simulink model "DC_MOTOR_CONTROL"  (R2022b)
settings: Solver=FixedStepAuto  StartTime=0.0  StopTime=100  FixedStep=0.01  RelTol=1e-3
libraries: fod x4, arduinolib x3, arduinosensorlib x1, SignalEditorBlockLib x1, simulink x1
settings Model: SimulationMode=external  ExtModeTrigDuration=2  Creator=Mario  LastModifiedBy=mario
settings DataIOCC: ReturnWorkspaceOutputs=off
settings OptimizationCC: EnhancedBackFolding=on  PassReuseOutputArgsThreshold=0  MaxStackSize=64  OptimizeBlockOrder=speed  DifferentSizesBufferReuse=on  OptimizationCustomize=off
settings DebuggingCC: ParameterTunabilityLossMsg=error
settings HardwareCC: ProdBitPerPointer=32  ProdBitPerSizeT=32  ProdBitPerPtrDiffT=32  ProdLargestAtomicInteger=Long  ProdLargestAtomicFloat=Double  ProdWordSize=32  ProdHWDeviceType=ARM Compatible->ARM Cortex  UseEmbeddedCoderFeatures=off
settings SFSimCC: MATLABDynamicMemAlloc=off
settings RTWCC: Description=Embedded Coder  SystemTargetFile=ert.tlc  HardwareBoard=Arduino Due  TLCOptions=-aInlineSetEventsForThisBaseRateFcn=TLC_FALSE -aSuppressMultiTaskScheduler=TLC_FALSE -aRateBasedStepFcn=1  TemplateMakefile=ert_default_tmf  Toolchain=Arduino ARM  BuildConfiguration=Faster Runs
settings CodeAppCC: ForceParamTrailComments=on  OperatorAnnotations=on
settings ERTTargetCC: ERTCustomFileBanners=off  SupportContinuousTime=on  SupportNonInlinedSFcns=on  RemoveResetFunc=off  SupportVariableSizeSignals=on  ModelStepFunctionPrototypeControlCompliant=off  ExtModeTransport=3  ExtModeStaticAlloc=on  ExtModeAutomaticAllocSize=off  ExtModeStaticAllocSize=24576  ExtModeMexFile=ext_xcp  ExtModeIntrfLevel=Level2 - Open

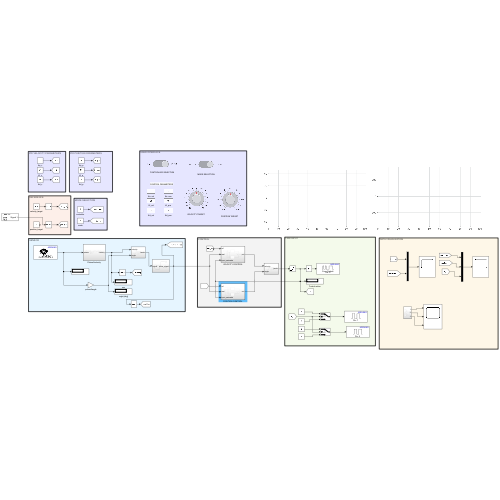
[thumbnail: Simulink's stored preview of the top-level diagram]
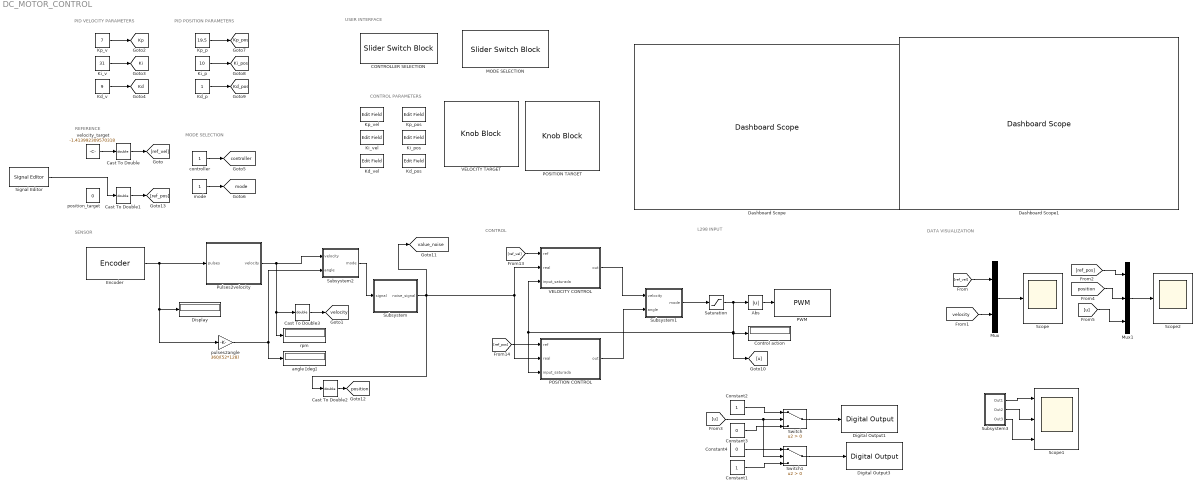
== system DC_MOTOR_CONTROL ==
  note: CONTROL PARAMETERS
  note: USER INTERFACE
  note: CONTROL
  note: MODE SELECTION
  note: DATA VISUALIZATION
  note: PID VELOCITY PARAMETERS
  note: SENSOR
  note: REFERENCE
  note: L298 INPUT
  note: PID POSITION PARAMETERS
  Abs : Abs  SaturateOnIntegerOverflow=off
  CONTROLLER SELECTION : SliderSwitchBlock  LabelPosition=Hide
      settings: Values={{'PID', 'FOPID'}, [0 1]}
  Cast To Double{,1..3} (4 alike) : DataTypeConversion  OutDataTypeStr=double  SaturateOnIntegerOverflow=off  RndMeth=Floor
  Constant1 : Constant
  Constant2 : Constant
  Constant3 : Constant  Value=0
  Constant4 : Constant  Value=0
  Control action : Display
  Dashboard Scope : DashboardScope  Ymin=-70  Ymax=70  UpdateMode=Scroll
  Dashboard Scope1 : DashboardScope  Ymin=-360  Ymax=360  UpdateMode=Scroll
  Digital Output1 : arduinolib/Digital Output  pinNumber=7  Direction=output  blockPlatform=arduino
  Digital Output3 : arduinolib/Digital Output  pinNumber=5  Direction=output  blockPlatform=arduino
  Display : Display
  Encoder : arduinosensorlib/Encoder  InputA=3  InputB=2  Mode=No reset  SampleTime=-1
  Kd_p : Constant
  Kd_pos : EditField  LabelPosition=Hide  ShowInitialText=on  Alignment=Center
  Kd_v : Constant  Value=9
  Kd_vel : EditField  LabelPosition=Hide  ShowInitialText=on  Alignment=Center
  Ki_p : Constant  Value=10
  Ki_pos : EditField  LabelPosition=Hide  ShowInitialText=on  Alignment=Center
  Ki_v : Constant  Value=31
  Ki_vel : EditField  LabelPosition=Hide  ShowInitialText=on  Alignment=Center
  Kp_p : Constant  Value=19.5
  Kp_pos : EditField  LabelPosition=Hide  ShowInitialText=on  Alignment=Center
  Kp_v : Constant  Value=7
  Kp_vel : EditField  LabelPosition=Hide  ShowInitialText=on  Alignment=Center
  MODE SELECTION : SliderSwitchBlock  LabelPosition=Hide
      settings: Values={{'Velocity', 'Position'}, [0 1]}
  Mux : Mux  Inputs=2
  Mux1 : Mux  Inputs=3
  POSITION CONTROL : Subsystem
  POSITION TARGET : KnobBlock  LabelPosition=Hide  ScaleMin=-360  ScaleMax=360
  PWM : arduinolib/PWM  pinNumber=8  frequencyType=Default  desiredFrequency=490.2  achievableFrequency=490.2
  Pulses2velocity : Subsystem
  Saturation : Saturate  UpperLimit=255  LowerLimit=-255
  Scope : Scope
  Scope1 : Scope  NumInputPorts=3
  Scope2 : Scope
  Signal Editor : SignalEditorBlockLib/Signal Editor  FileName=ANGLE_REFERENCE.mat  ActiveScenario=Scenario  ActiveSignal=Signal 1  IsBus=off  OutputBusObjectStr=Bus: BusObject  SampleTime=0  Interpolate=off  ZeroCross=off  OutputAfterFinalValue=Setting to zero  Unit=inherit  PreserveSignalName=on
  Subsystem : Subsystem
  Subsystem1 : Subsystem
  Subsystem2 : Subsystem
  Subsystem3 : Subsystem
  Switch : Switch  Criteria=u2 > Threshold  SaturateOnIntegerOverflow=off  InputSameDT=off
  Switch1 : Switch  Criteria=u2 > Threshold  SaturateOnIntegerOverflow=off  InputSameDT=off
  VELOCITY CONTROL : Subsystem
  VELOCITY TARGET : KnobBlock  LabelPosition=Hide  ScaleMin=-70  ScaleMax=70
  angle [deg] : Display
  controller : Constant
  mode : Constant
  position_target : Constant  Value=0
  pulses2angle : Gain  Gain=360/(52*128)
  rpm : Display
  velocity_target : Constant  Value=-1.413992309570318
  tag scope: Kd=global, Kd_pos=global, Ki=global, Ki_pos=global, Kp=global, Kp_pos=global, controller=global, mode=global, position=global, value_noise=global, velocity=global
  wires:
  Constant3/1 -> Switch/3
  Constant2/1 -> Switch/1
  Switch/1 -> Digital Output1/1
  Switch1/1 -> Digital Output3/1
  Pulses2velocity/1(velocity) -> Subsystem2/1(velocity), rpm/1, Cast To Double3/1
  velocity_target/1 -> Cast To Double/1
  Encoder/1 -> Pulses2velocity/1(pulses), pulses2angle/1, Display/1
  Saturation/1 -> POSITION CONTROL/3(input_saturada), VELOCITY CONTROL/3(input_saturada), [u], Control action/1, Abs/1
  Constant4/1 -> Switch1/1
  Constant1/1 -> Switch1/3
  [ref_vel] -> Mux/1
  [velocity] -> Mux/2
  Kp_v/1 -> [Kp]
  Ki_v/1 -> [Ki]
  Kd_v/1 -> [Kd]
  controller/1 -> [controller]
  mode/1 -> [mode]
  VELOCITY CONTROL/1(out) -> Subsystem1/1(velocity)
  POSITION CONTROL/1(out) -> Subsystem1/2(angle)
  pulses2angle/1 -> Subsystem2/2(angle), angle [deg]/1
  Kp_p/1 -> [Kp_pos]
  Kd_p/1 -> [Kd_pos]
  Ki_p/1 -> [Ki_pos]
  Mux/1 -> Scope/1
  Abs/1 -> PWM/1
  [u] -> Switch/2, Switch1/2
  Subsystem2/1(mode) -> Subsystem/1(signal)
  [ref_vel] -> VELOCITY CONTROL/1(ref)
  [ref_pos] -> POSITION CONTROL/1(ref)
  Subsystem3/1(Out1) -> Scope1/1
  Subsystem3/2(Out2) -> Scope1/2
  Subsystem3/3(Out3) -> Scope1/3
  Subsystem/1(noise_signal) -> Cast To Double2/1, POSITION CONTROL/2(real), VELOCITY CONTROL/2(real), [value_noise]
  Mux1/1 -> Scope2/1
  [ref_pos] -> Mux1/1
  [position] -> Mux1/2
  Cast To Double/1 -> [ref_vel]
  Cast To Double1/1 -> [ref_pos]
  Cast To Double2/1 -> [position]
  Cast To Double3/1 -> [velocity]
  Signal Editor/1 -> Cast To Double1/1
  [u] -> Mux1/3
  Subsystem1/1(mode) -> Saturation/1

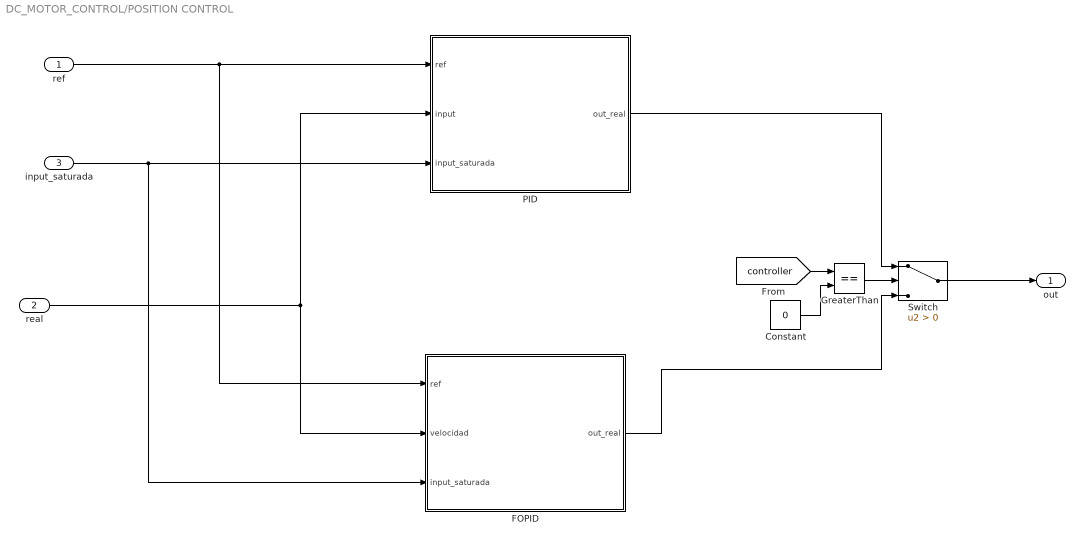
== system DC_MOTOR_CONTROL/POSITION CONTROL ==
  ref : Inport
  real : Inport  Port=2
  input_saturada : Inport  Port=3
  Constant : Constant  Value=0
  "FOPID " : Subsystem
  GreaterThan : RelationalOperator  Operator===  OutDataTypeStr=boolean  RndMeth=Simplest  InputSameDT=off
  PID : Subsystem
  Switch : Switch  Criteria=u2 > Threshold  SaturateOnIntegerOverflow=off  InputSameDT=off
  out : Outport
  wires:
  input_saturada/1 -> "FOPID "/3(input_saturada), PID/3(input_saturada)
  ref/1 -> "FOPID "/1(ref), PID/1(ref)
  real/1 -> "FOPID "/2(velocidad), PID/2(input)
  "FOPID "/1(out_real) -> Switch/3
  PID/1(out_real) -> Switch/1
  Switch/1 -> out/1
  [controller] -> GreaterThan/1
  Constant/1 -> GreaterThan/2
  GreaterThan/1 -> Switch/2

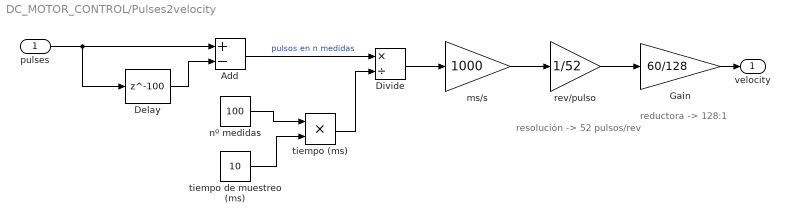
== system DC_MOTOR_CONTROL/Pulses2velocity ==
  note: reductora -> 128:1
  note: resolución -> 52 pulsos/rev
  pulses : Inport
  Add : Sum  Inputs=+-
  Delay : Delay  DelayLength=100
  Divide : Product  Inputs=*/
  Gain : Gain  Gain=60/128
  ms/s : Gain  Gain=1000
  nº medidas : Constant  Value=100
  rev/pulso : Gain  Gain=1/52
  tiempo (ms) : Product  Inputs=**
  tiempo de muestreo (ms) : Constant  Value=10
  velocity : Outport
  wires:
  Delay/1 -> Add/2
  Divide/1 -> ms/s/1
  pulses/1 -> Delay/1, Add/1
  nº medidas/1 -> tiempo (ms)/1
  Add/1 -> Divide/1  "pulsos en n medidas"
  rev/pulso/1 -> Gain/1
  Gain/1 -> velocity/1
  ms/s/1 -> rev/pulso/1
  tiempo de muestreo (ms)/1 -> tiempo (ms)/2
  tiempo (ms)/1 -> Divide/2

== system DC_MOTOR_CONTROL/Subsystem ==
  signal : Inport
  Band-Limited White Noise : simulink/Sources/Band-Limited White Noise  Cov=0  Ts=0.01  seed=[23341]
  Sum : Sum  Inputs=|++
  noise_signal : Outport
  wires:
  Sum/1 -> noise_signal/1
  signal/1 -> Sum/2
  Band-Limited White Noise/1 -> Sum/1

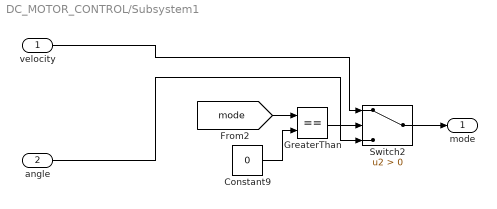
== system DC_MOTOR_CONTROL/Subsystem1 ==
  velocity : Inport
  angle : Inport  Port=2
  Constant9 : Constant  Value=0
  GreaterThan : RelationalOperator  Operator===  OutDataTypeStr=boolean  RndMeth=Simplest  InputSameDT=off
  Switch2 : Switch  Criteria=u2 > Threshold  SaturateOnIntegerOverflow=off  InputSameDT=off
  mode : Outport
  wires:
  [mode] -> GreaterThan/1
  GreaterThan/1 -> Switch2/2
  Switch2/1 -> mode/1
  Constant9/1 -> GreaterThan/2
  velocity/1 -> Switch2/1
  angle/1 -> Switch2/3

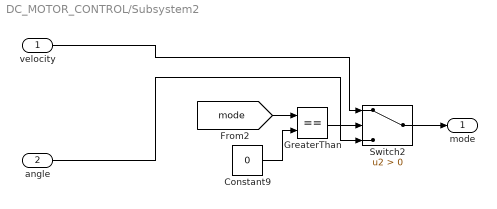
== system DC_MOTOR_CONTROL/Subsystem2 ==
  velocity : Inport
  angle : Inport  Port=2
  Constant9 : Constant  Value=0
  GreaterThan : RelationalOperator  Operator===  OutDataTypeStr=boolean  RndMeth=Simplest  InputSameDT=off
  Switch2 : Switch  Criteria=u2 > Threshold  SaturateOnIntegerOverflow=off  InputSameDT=off
  mode : Outport
  wires:
  [mode] -> GreaterThan/1
  GreaterThan/1 -> Switch2/2
  Switch2/1 -> mode/1
  Constant9/1 -> GreaterThan/2
  velocity/1 -> Switch2/1
  angle/1 -> Switch2/3

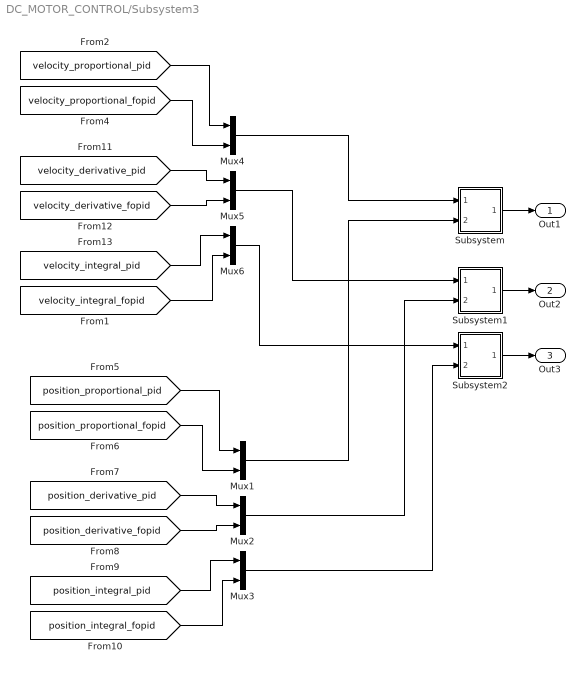
== system DC_MOTOR_CONTROL/Subsystem3 ==
  Mux{1..6} (6 alike) : Mux  Inputs=2
  Subsystem : Subsystem
  Subsystem1 : Subsystem
  Subsystem2 : Subsystem
  Out1 : Outport
  Out2 : Outport  Port=2
  Out3 : Outport  Port=3
  wires:
  [position_proportional_fopid] -> Mux1/2
  [position_derivative_pid] -> Mux2/1
  [position_proportional_pid] -> Mux1/1
  [position_derivative_fopid] -> Mux2/2
  [position_integral_pid] -> Mux3/1
  [position_integral_fopid] -> Mux3/2
  [velocity_proportional_fopid] -> Mux4/2
  [velocity_integral_pid] -> Mux6/1
  [velocity_derivative_fopid] -> Mux5/2
  [velocity_integral_fopid] -> Mux6/2
  [velocity_proportional_pid] -> Mux4/1
  [velocity_derivative_pid] -> Mux5/1
  Mux4/1 -> Subsystem/1(In1)
  Mux1/1 -> Subsystem/2(In2)
  Mux5/1 -> Subsystem1/1(In1)
  Mux2/1 -> Subsystem1/2(In2)
  Mux6/1 -> Subsystem2/1(In1)
  Mux3/1 -> Subsystem2/2(In2)
  Subsystem/1(Out1) -> Out1/1
  Subsystem1/1(Out1) -> Out2/1
  Subsystem2/1(Out1) -> Out3/1

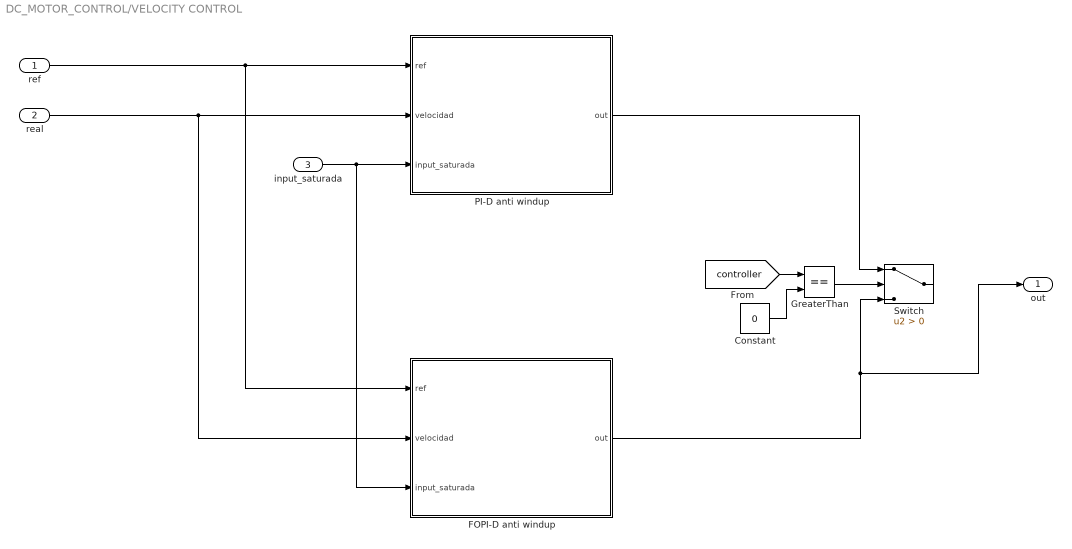
== system DC_MOTOR_CONTROL/VELOCITY CONTROL ==
  ref : Inport
  real : Inport  Port=2
  input_saturada : Inport  Port=3
  Constant : Constant  Value=0
  FOPI-D anti windup : Subsystem
  GreaterThan : RelationalOperator  Operator===  OutDataTypeStr=boolean  RndMeth=Simplest  InputSameDT=off
  PI-D anti windup : Subsystem
  Switch : Switch  Criteria=u2 > Threshold  SaturateOnIntegerOverflow=off  InputSameDT=off
  out : Outport
  wires:
  input_saturada/1 -> PI-D anti windup/3(input_saturada), FOPI-D anti windup/3(input_saturada)
  PI-D anti windup/1(out) -> Switch/1
  [controller] -> GreaterThan/1
  Constant/1 -> GreaterThan/2
  GreaterThan/1 -> Switch/2
  FOPI-D anti windup/1(out) -> out/1, Switch/3
  ref/1 -> PI-D anti windup/1(ref), FOPI-D anti windup/1(ref)
  real/1 -> PI-D anti windup/2(velocidad), FOPI-D anti windup/2(velocidad)

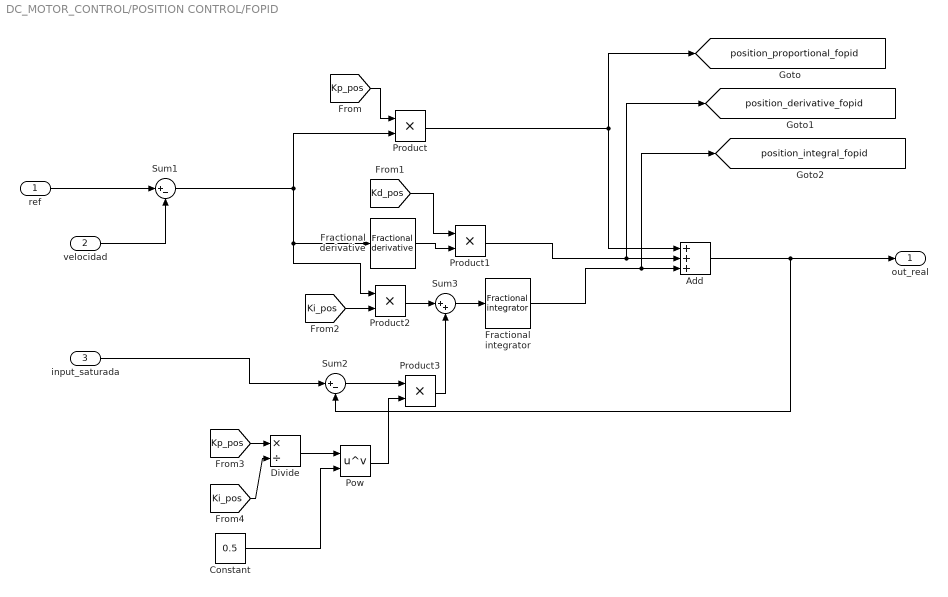
== system DC_MOTOR_CONTROL/POSITION CONTROL/FOPID  ==
  ref : Inport
  velocidad : Inport  Port=2
  input_saturada : Inport  Port=3
  Add : Sum  Inputs=+++
  Constant : Constant  Value=0.5
  Divide : Product  Inputs=*/
  Fractional derivative : fod/Fractional derivative  gam=0.95  ww=[0.1; 50]  n=5  nFod=off
      settings: SourceProductName=FOMCON Toolbox
  Fractional integrator : fod/Fractional integrator  gam=0.15  ww=[0.1; 50]  n=5  nFod=off
      settings: SourceProductName=FOMCON Toolbox
  Pow : Math  Operator=pow  SignedPower=on  RndMeth=Zero
  Product{,1..3} (4 alike) : Product
  Sum1 : Sum  Inputs=|+-
  Sum2 : Sum  Inputs=|+-
  Sum3 : Sum  Inputs=|++
  out_real : Outport
  tag scope: position_derivative_fopid=global, position_integral_fopid=global, position_proportional_fopid=global
  wires:
  ref/1 -> Sum1/1
  velocidad/1 -> Sum1/2
  Add/1 -> Sum2/2, out_real/1
  Sum1/1 -> Product2/1, Fractional derivative/1, Product/2
  Product2/1 -> Sum3/1
  Sum3/1 -> Fractional integrator/1
  Sum2/1 -> Product3/1
  input_saturada/1 -> Sum2/1
  Fractional derivative/1 -> Product1/2
  [Kp_pos] -> Product/1
  [Kd_pos] -> Product1/1
  [Ki_pos] -> Product2/2
  [Kp_pos] -> Divide/1
  [Ki_pos] -> Divide/2
  Divide/1 -> Pow/1
  Constant/1 -> Pow/2
  Pow/1 -> Product3/2
  Product3/1 -> Sum3/2
  Fractional integrator/1 -> [position_integral_fopid], Add/3
  Product/1 -> Add/1, [position_proportional_fopid]
  Product1/1 -> [position_derivative_fopid], Add/2

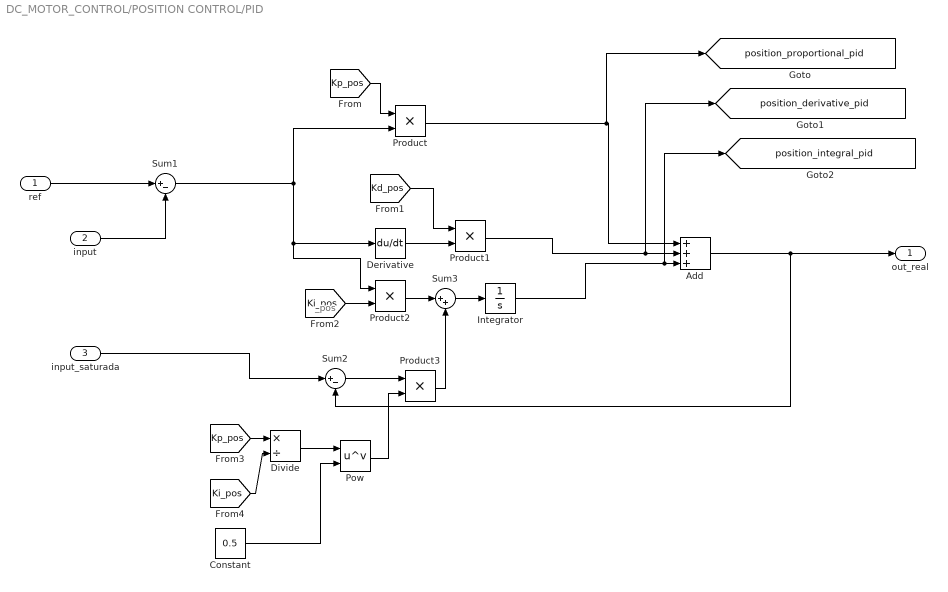
== system DC_MOTOR_CONTROL/POSITION CONTROL/PID ==
  note: _pos
  ref : Inport
  input : Inport  Port=2
  input_saturada : Inport  Port=3
  Add : Sum  Inputs=+++
  Constant : Constant  Value=0.5
  Derivative : Derivative
  Divide : Product  Inputs=*/
  Integrator : Integrator
  Pow : Math  Operator=pow  SignedPower=on  RndMeth=Zero
  Product{,1..3} (4 alike) : Product
  Sum1 : Sum  Inputs=|+-
  Sum2 : Sum  Inputs=|+-
  Sum3 : Sum  Inputs=|++
  out_real : Outport
  tag scope: position_derivative_pid=global, position_integral_pid=global, position_proportional_pid=global
  wires:
  ref/1 -> Sum1/1
  input/1 -> Sum1/2
  Add/1 -> Sum2/2, out_real/1
  Product/1 -> [position_proportional_pid], Add/1
  Sum1/1 -> Product2/1, Derivative/1, Product/2
  Product1/1 -> Add/2, [position_derivative_pid]
  Product2/1 -> Sum3/1
  Sum3/1 -> Integrator/1
  Sum2/1 -> Product3/1
  Integrator/1 -> [position_integral_pid], Add/3
  input_saturada/1 -> Sum2/1
  Derivative/1 -> Product1/2
  [Kp_pos] -> Product/1
  [Kd_pos] -> Product1/1
  [Ki_pos] -> Product2/2
  [Kp_pos] -> Divide/1
  [Ki_pos] -> Divide/2
  Divide/1 -> Pow/1
  Constant/1 -> Pow/2
  Pow/1 -> Product3/2
  Product3/1 -> Sum3/2

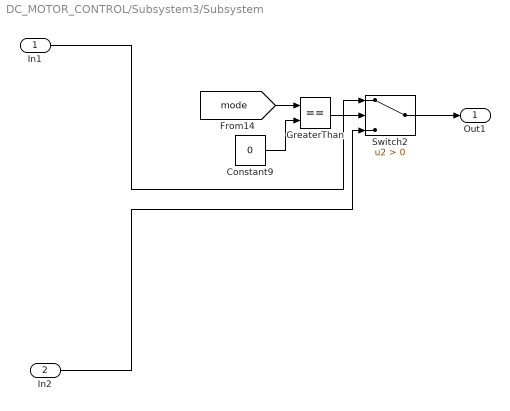
== system DC_MOTOR_CONTROL/Subsystem3/Subsystem ==
  In1 : Inport
  In2 : Inport  Port=2
  Constant9 : Constant  Value=0
  GreaterThan : RelationalOperator  Operator===  OutDataTypeStr=boolean  RndMeth=Simplest  InputSameDT=off
  Switch2 : Switch  Criteria=u2 > Threshold  SaturateOnIntegerOverflow=off  InputSameDT=off
  Out1 : Outport
  wires:
  Constant9/1 -> GreaterThan/2
  In2/1 -> Switch2/3
  [mode] -> GreaterThan/1
  In1/1 -> Switch2/1
  GreaterThan/1 -> Switch2/2
  Switch2/1 -> Out1/1

== system DC_MOTOR_CONTROL/Subsystem3/Subsystem1 ==
  In1 : Inport
  In2 : Inport  Port=2
  Constant9 : Constant  Value=0
  GreaterThan : RelationalOperator  Operator===  OutDataTypeStr=boolean  RndMeth=Simplest  InputSameDT=off
  Switch2 : Switch  Criteria=u2 > Threshold  SaturateOnIntegerOverflow=off  InputSameDT=off
  Out1 : Outport
  wires:
  Constant9/1 -> GreaterThan/2
  In2/1 -> Switch2/3
  [mode] -> GreaterThan/1
  In1/1 -> Switch2/1
  GreaterThan/1 -> Switch2/2
  Switch2/1 -> Out1/1

== system DC_MOTOR_CONTROL/Subsystem3/Subsystem2 ==
  In1 : Inport
  In2 : Inport  Port=2
  Constant9 : Constant  Value=0
  GreaterThan : RelationalOperator  Operator===  OutDataTypeStr=boolean  RndMeth=Simplest  InputSameDT=off
  Switch2 : Switch  Criteria=u2 > Threshold  SaturateOnIntegerOverflow=off  InputSameDT=off
  Out1 : Outport
  wires:
  Constant9/1 -> GreaterThan/2
  In2/1 -> Switch2/3
  [mode] -> GreaterThan/1
  In1/1 -> Switch2/1
  GreaterThan/1 -> Switch2/2
  Switch2/1 -> Out1/1

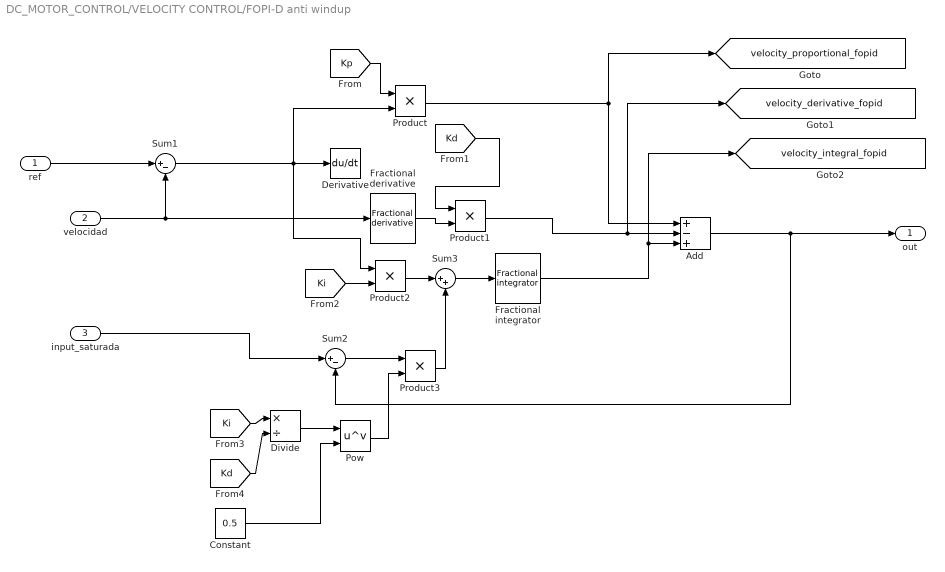
== system DC_MOTOR_CONTROL/VELOCITY CONTROL/FOPI-D anti windup ==
  ref : Inport
  velocidad : Inport  Port=2
  input_saturada : Inport  Port=3
  Add : Sum  Inputs=+-+
  Constant : Constant  Value=0.5
  Derivative : Derivative
  Divide : Product  Inputs=*/
  Fractional derivative : fod/Fractional derivative  gam=0.75  ww=[0.001; 50]  n=5  nFod=off
      settings: SourceProductName=FOMCON Toolbox
  Fractional integrator : fod/Fractional integrator  gam=0.75  ww=[0.001; 50]  n=5  nFod=off
      settings: SourceProductName=FOMCON Toolbox
  Pow : Math  Operator=pow  SignedPower=on  RndMeth=Zero
  Product{,1..3} (4 alike) : Product
  Sum1 : Sum  Inputs=|+-
  Sum2 : Sum  Inputs=|+-
  Sum3 : Sum  Inputs=|++
  out : Outport
  tag scope: velocity_derivative_fopid=global, velocity_integral_fopid=global, velocity_proportional_fopid=global
  wires:
  ref/1 -> Sum1/1
  velocidad/1 -> Fractional derivative/1, Sum1/2
  Add/1 -> Sum2/2, out/1
  Sum1/1 -> Product2/1, Derivative/1, Product/2
  Product2/1 -> Sum3/1
  Sum3/1 -> Fractional integrator/1
  Sum2/1 -> Product3/1
  input_saturada/1 -> Sum2/1
  Fractional derivative/1 -> Product1/2
  [Kp] -> Product/1
  [Kd] -> Product1/1
  [Ki] -> Product2/2
  [Ki] -> Divide/1
  [Kd] -> Divide/2
  Divide/1 -> Pow/1
  Constant/1 -> Pow/2
  Pow/1 -> Product3/2
  Product3/1 -> Sum3/2
  Product1/1 -> [velocity_derivative_fopid], Add/2
  Product/1 -> Add/1, [velocity_proportional_fopid]
  Fractional integrator/1 -> [velocity_integral_fopid], Add/3

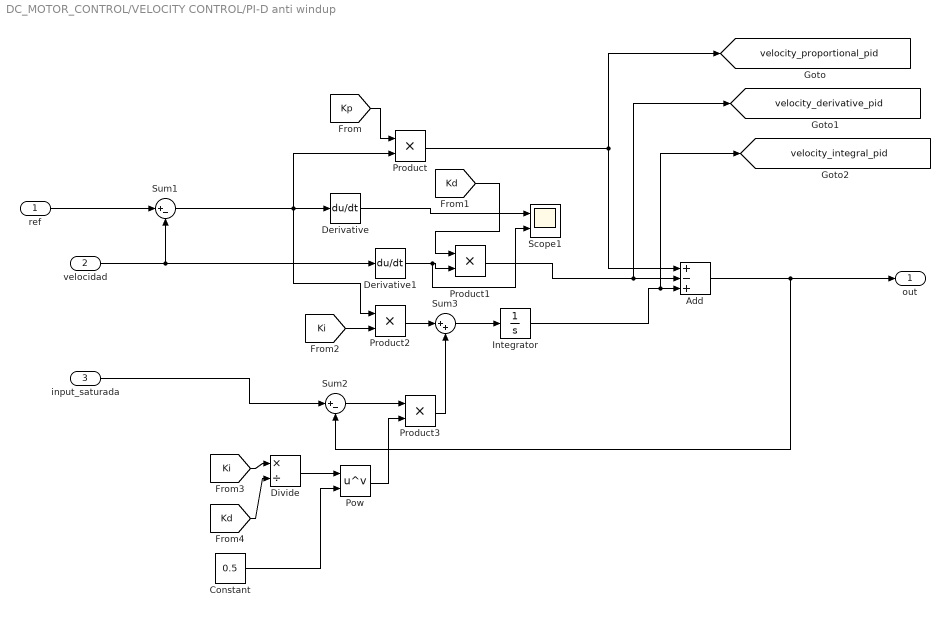
== system DC_MOTOR_CONTROL/VELOCITY CONTROL/PI-D anti windup ==
  ref : Inport
  velocidad : Inport  Port=2
  input_saturada : Inport  Port=3
  Add : Sum  Inputs=+-+
  Constant : Constant  Value=0.5
  Derivative : Derivative
  Derivative1 : Derivative
  Divide : Product  Inputs=*/
  Integrator : Integrator
  Pow : Math  Operator=pow  SignedPower=on  RndMeth=Zero
  Product{,1..3} (4 alike) : Product
  Scope1 : Scope  NumInputPorts=2
  Sum1 : Sum  Inputs=|+-
  Sum2 : Sum  Inputs=|+-
  Sum3 : Sum  Inputs=|++
  out : Outport
  tag scope: velocity_derivative_pid=global, velocity_integral_pid=global, velocity_proportional_pid=global
  wires:
  ref/1 -> Sum1/1
  velocidad/1 -> Derivative1/1, Sum1/2
  Add/1 -> Sum2/2, out/1
  Sum1/1 -> Product2/1, Derivative/1, Product/2
  Product2/1 -> Sum3/1
  Sum3/1 -> Integrator/1
  Sum2/1 -> Product3/1
  input_saturada/1 -> Sum2/1
  Derivative1/1 -> Scope1/2, Product1/2
  [Kp] -> Product/1
  [Kd] -> Product1/1
  [Ki] -> Product2/2
  [Ki] -> Divide/1
  [Kd] -> Divide/2
  Divide/1 -> Pow/1
  Constant/1 -> Pow/2
  Pow/1 -> Product3/2
  Product3/1 -> Sum3/2
  Derivative/1 -> Scope1/1
  Product1/1 -> [velocity_derivative_pid], Add/2
  Product/1 -> [velocity_proportional_pid], Add/1
  Integrator/1 -> [velocity_integral_pid], Add/3
